simulink model "FIR_InterpolationStream_Ex1"  (R2023a)
settings: Solver=VariableStepAuto  StartTime=0.0  StopTime=1  RelTol=1e-3
PostLoadFcn:
  | Fs = 50e3;               % Sampling Frequency
  | Fpass = 16000;            % Passband Frequency
  | Fstop = 23000;            % Stopband Frequency
  | Dpass = 0.00460513763;    % Passband Ripple
  | Dstop = 0.0001;           % Stopband Attenuation
  | dens  = 16;                   % Density Factor
  | % Calculate the order from the parameters using FIRPMORD.
  | [N, Fo, Ao, W] = firpmord([Fpass, Fstop]/(Fs/2), [1 0], [Dpass, Dstop]);
  | % Calculate the coefficients using the FIRPM function.
  | b  = firpm(N, Fo, Ao, W, {dens});
  | coeffs = b;
undefined symbols (not defined in the file): FIR_InterpolationStream_FilterCoeffs, None, S, vsva2197, xcvc1902
libraries: dspsrcs4 x1, aieDSP x1, dspmlti4 x1, vmcUtilities x1
settings Model: Creator=sdegala  LastModifiedBy=robg
settings ModelReferenceCC: EnableRefExpFcnMdlSchedulingChecks=on

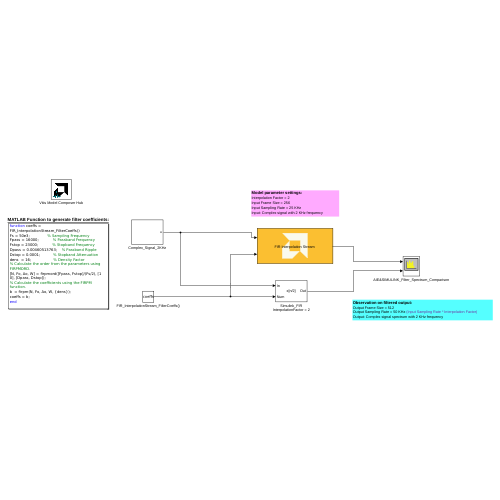
[thumbnail: Simulink's stored preview of the top-level diagram]
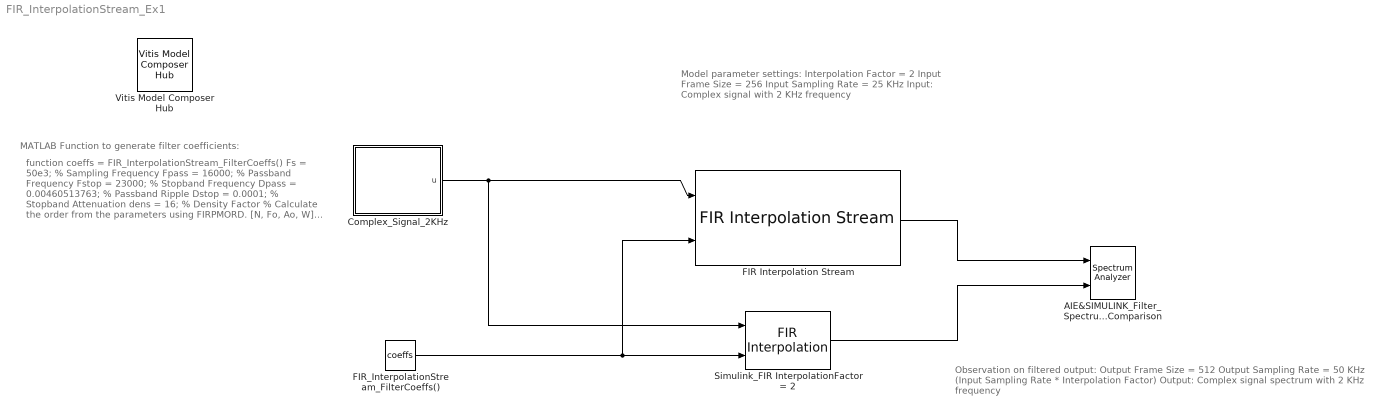
== system FIR_InterpolationStream_Ex1 ==
  note: Observation on filtered output:
      | Output Frame Size = 512
      | Output Sampling Rate = 50 KHz (Input Sampling Rate * Interpolation Factor)
      | Output: Complex signal spectrum with 2 KHz frequency
  note: MATLAB Function to generate filter coefficients:
  note: function coeffs = FIR_InterpolationStream_FilterCoeffs()
      | Fs = 50e3; % Sampling Frequency
      | Fpass = 16000; % Passband Frequency
      | Fstop = 23000; % Stopband Frequency
      | Dpass = 0.00460513763; % Passband Ripple
      | Dstop = 0.0001; % Stopband Attenuation
      | dens = 16; % Density Factor
      | % Calculate the order from the parameters using FIRPMORD.
      | [N, Fo, Ao, W] = firpmord([Fpass, Fstop]/(Fs/2), [1 0], [Dpass, Dstop]);
      | % Calculate the coefficients using the FIRPM function.
      | b = firpm(N, Fo, Ao, W, {dens});
      | coeffs = b;
      | end
  note: Model parameter settings:
      | Interpolation Factor = 2
      | Input Frame Size = 256
      | Input Sampling Rate = 25 KHz
      | Input: Complex signal with 2 KHz frequency
  AIE&SIMULINK_Filter_Spectrum_Comparison : SpectrumAnalyzer  NumInputPorts=2  AveragingMethod=Exponential  ShowLegend=on  ChannelNames="[\"\"]"  DefaultConfigurationName=spbscopes.SpectrumAnalyzerBlockCfg
  Complex_Signal_2KHz : Subsystem
  FIR Interpolation Stream : aieDSP/FIR Interpolation Stream  data_type=cfloat  coef_type=float  use_coeff_reload=on  dual_ip=off  num_outputs=off  coeff=FIR_InterpolationStream_FilterCoeffs()  fir_length=24  interpolate_factor=2  input_window_size=256  shift_val=0  rnd_mode=Round to positive infinity  sat_mode=0-None  ssr=1  interp_poly=1  casc_length=1  AIE_VARIANT=1  blockJsonConstraints=[]  blockJsonConstraintsInternal=[]  spec=vmc_stream_fir_interpolate_asym.json  SerializedMaskParamNames=[]  SerializedMaskParamValues=[]  SerializedMaskParamVisibilities=[]  block_type=FIR Interpolation Stream  SerializedMaskParamDataypes=typename|typename|bool|bool|bool|coef_type|uint|uint|uint|uint|uint|uint|uint|uint|uint|uint  SerializedMaskParamEnumStrArr=0|0|0|0|0|0|0|0|0|0|Floor,Ceiling,Round to positive infinity,Round to negative infinity,Round symmetrical to infinity,Round symmetrical to zero,Round convergent to even,Round convergent to odd|0-None,1-Asymmetric,3-Symmetric|0|0|0|0  SerializedMaskParamEnumValArr=0|0|0|0|0|0|0|0|0|0|0,1,2,3,4,5,6,7|0,1,3|0|0|0|0  SerializedMaskParamVectorArr=0|0|0|0|0|1|0|0|0|0|0|0|0|0|0|0
  FIR_InterpolationStream_FilterCoeffs() : Constant  Value=coeffs  OutDataTypeStr=single
  Simulink_FIR InterpolationFactor = 2 : dspmlti4/FIR Interpolation  FilterSource=Input port  PrivateCoeffs=0  h=coeffs  L=2  FilterObject=FINTERP  InputProcessing=Columns as channels (frame based)  framing=Enforce single-rate processing  outputBufInitCond=0  roundingMode=Ceiling  overflowMode=off  firstCoeffDataTypeStr=Inherit: Same word length as input  firstCoeffMin=[]  firstCoeffMax=[]  firstCoeffLastDataTypeStr=Inherit: Same word length as input  outputMin=[]  outputMax=[]
  Vitis Model Composer Hub : vmcUtilities/Vitis Model Composer Hub  Tag=genX  CodeGeneration=off  StartColumn=1  NumberOfColumns=1  TargetDirectory=./code  exportDesign=off  analyzeDesign=off  validateDesignOnHw=off  ExportType=AI Engines  IpVendor=xilinx.com  IpLibrary=hls  IpVersion=1.0  IpHWLanguage=Verilog  AieCompilerOptions={}  AieSimulatorOptions={}  CreateTestbench=off  TestbenchStackSize=10  RunRtlSim=off  RunCSim=off  RunAieSim=off  AieSimTimeout=50000  RunAieSimProfiling=off  LaunchVitisAnalyzer=off  PlotOutput=off  RunX86Sim=off  X86SimTimeout=10  GenHwImage=off  GenLibadfXo=off  GenHwValidationCode=off  PlatformType=Not Specified  HwSystemType=Baremetal  HwValidationTarget=hw  ProjDevice=xcvc1902-vsva2197-1LP-e-S  ProjDevicePart=xcvc1902-vsva2197-1LP-e-S  AIEType=AIE  SamplePeriod=-1  ClockFrequency=200  DataPathParallelism=1  xilinxfamily=versalaicore  part=xcvc1902  speed=-1LP-e-S  package=vsva2197  directory=./netlist  testbench=off  incr_netlist=off  synthesis_tool=Vivado  clock_wrapper=Clock Enables  dbl_ovrd=According to Block Masks  dcm_input_clock_period=10  sysclk_period=10  simulink_period=1  eval_field=0  LogFileName=''  NThreads=4
  wires:
  FIR_InterpolationStream_FilterCoeffs()/1 -> Simulink_FIR InterpolationFactor = 2/2, FIR Interpolation Stream/2
  Simulink_FIR InterpolationFactor = 2/1 -> AIE&SIMULINK_Filter_Spectrum_Comparison/2
  Complex_Signal_2KHz/1(u) -> FIR Interpolation Stream/1, Simulink_FIR InterpolationFactor = 2/1
  FIR Interpolation Stream/1 -> AIE&SIMULINK_Filter_Spectrum_Comparison/1

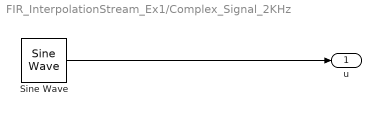
== system FIR_InterpolationStream_Ex1/Complex_Signal_2KHz ==
  Sine Wave : dspsrcs4/Sine Wave  Amplitude=1  Frequency=2e3  Phase=0  SampleMode=Discrete  OutComplex=Complex  CompMethod=Trigonometric fcn  TableSize=Speed  SampleTime=1/25e3  SamplesPerFrame=256  ResetState=Restart at time zero  OutputFrames=off  dataType=single  wordLen=16  udDataType=sfix(16)  fracBitsMode=Best precision  numFracBits=15  OutDataTypeStr=single  LastOutDataTypeStr=single
  u : Outport
  wires:
  Sine Wave/1 -> u/1
